simulink model "step1_TrajectoryPlanningModel"  (Simulink 10.2)
settings: Solver=VariableStepAuto  StartTime=0.0  StopTime=10.0  RelTol=1e-3
values from neighbouring files (symbols this model uses):
  L0 = z(7)    [Forward_kinematics.m]    (also in GeometricCalculation_simulink.m = Geoparams(4); PRBDM_3R_parameters.m = 0.03; PRBDM_3R_parameters.mat = 0.03; TrajectoryPlanning_simulink.m = X(8))
  L1 = z(8)    [Forward_kinematics.m]    (also in GeometricCalculation_simulink.m = Geoparams(5); Jacobi.m = x(4); PRBDM_3R_CTC.m = x(19); PRBDM_3R_Dynamic_Matrices_NewtonEular.m = robot_params(4))
  L2 = z(9)    [Forward_kinematics.m]    (also in GeometricCalculation_simulink.m = Geoparams(6); Jacobi.m = x(5); PRBDM_3R_CTC.m = x(20); PRBDM_3R_Dynamic_Matrices_NewtonEular.m = robot_params(5))
  L3 = z(10)    [Forward_kinematics.m]    (also in GeometricCalculation_simulink.m = Geoparams(7); Jacobi.m = x(6); PRBDM_3R_CTC.m = x(21); PRBDM_3R_Dynamic_Matrices_NewtonEular.m = robot_params(6))
  phi = pi/3    (= 1.0471975512)    [PRBDM_3R_test001.m]
  xd = 0.0536    [PRBDM_3R_test001.m]    (also in PRBDM_CTC_task.m = z(13); RRR_CTC_task.m = z(13))
  yd = 0.0135    [PRBDM_3R_test001.m]    (also in PRBDM_CTC_task.m = z(14); RRR_CTC_task.m = z(14))
settings Model: Creator=Master  LastModifiedBy=Master
settings DataIOCC: SaveFormat=Dataset  SignalLoggingSaveFormat=Dataset  ReturnWorkspaceOutputs=on
settings OptimizationCC: LifeSpan=auto
settings DebuggingCC: UnderspecifiedInitializationDetection=Simplified  MergeDetectMultiDrivingBlocksExec=error  FcnCallInpInsideContextMsg=error  SFUnexpectedBacktrackingDiag=error  SFNoUnconditionalDefaultTransitionDiag=error  SFExecutionAtInitializationDiag=warning  UnderSpecifiedDimensionMsg=error  ArithmeticOperatorsInVariantConditions=error
settings HardwareCC: ProdBitPerPointer=64  ProdBitPerSizeT=64  ProdBitPerPtrDiffT=64  ProdLargestAtomicFloat=Float  ProdIntDivRoundTo=Zero  ProdEndianess=LittleEndian  ProdWordSize=64  ProdHWDeviceType=Intel->x86-64 (Windows64)
settings ModelReferenceCC: PropagateSignalLabelsOutOfModel=on
settings SFSimCC: SimUseLocalCustomCode=on  CustomCodeUndefinedFunction=FilterOut
settings RTWCC: RTWUseLocalCustomCode=on
settings CodeAppCC: StateflowObjectComments=off
settings GRTTargetCC: TargetLangStandard=C99 (ISO)  CombineOutputUpdateFcns=on  GRTInterface=off
settings ConfigComp: CovMetricSettings=dwe  CovSaveCumulativeToWorkspaceVar=off  CovSaveSingleToWorkspaceVar=off  CovExternalEMLEnable=on

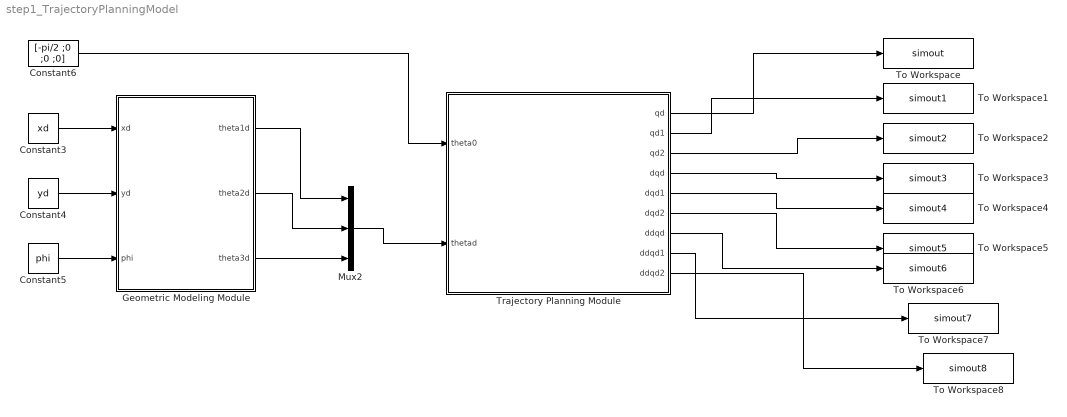
== system step1_TrajectoryPlanningModel ==
  Constant3 : Constant  Value=xd
  Constant4 : Constant  Value=yd
  Constant5 : Constant  Value=phi
  Constant6 : Constant  Value=[-pi/2 ;0 ;0 ;0]
  Geometric Modeling Module : Subsystem
  Mux2 : Mux  Inputs=3
  To Workspace : ToWorkspace  VariableName=simout  SaveFormat=Timeseries  SampleTime=-1
  To Workspace1 : ToWorkspace  VariableName=simout1  SaveFormat=Timeseries  SampleTime=-1
  To Workspace2 : ToWorkspace  VariableName=simout2  SaveFormat=Timeseries  SampleTime=-1
  To Workspace3 : ToWorkspace  VariableName=simout3  SaveFormat=Timeseries  SampleTime=-1
  To Workspace4 : ToWorkspace  VariableName=simout4  SaveFormat=Timeseries  SampleTime=-1
  To Workspace5 : ToWorkspace  VariableName=simout5  SaveFormat=Timeseries  SampleTime=-1
  To Workspace6 : ToWorkspace  VariableName=simout6  SaveFormat=Timeseries  SampleTime=-1
  To Workspace7 : ToWorkspace  VariableName=simout7  SaveFormat=Timeseries  SampleTime=-1
  To Workspace8 : ToWorkspace  VariableName=simout8  SaveFormat=Timeseries  SampleTime=-1
  Trajectory Planning Module : Subsystem
  wires:
  Constant4/1 -> Geometric Modeling Module/2(yd)
  Constant5/1 -> Geometric Modeling Module/3(phi)
  Constant3/1 -> Geometric Modeling Module/1(xd)
  Geometric Modeling Module/1(theta1d) -> Mux2/1
  Geometric Modeling Module/2(theta2d) -> Mux2/2
  Geometric Modeling Module/3(theta3d) -> Mux2/3
  Mux2/1 -> Trajectory Planning Module/2(thetad)
  Constant6/1 -> Trajectory Planning Module/1(theta0)
  Trajectory Planning Module/7(ddqd) -> To Workspace6/1
  Trajectory Planning Module/4(dqd) -> To Workspace3/1
  Trajectory Planning Module/3(qd2) -> To Workspace2/1
  Trajectory Planning Module/5(dqd1) -> To Workspace4/1
  Trajectory Planning Module/2(qd1) -> To Workspace1/1
  Trajectory Planning Module/6(dqd2) -> To Workspace5/1
  Trajectory Planning Module/8(ddqd1) -> To Workspace7/1
  Trajectory Planning Module/9(ddqd2) -> To Workspace8/1
  Trajectory Planning Module/1(qd) -> To Workspace/1

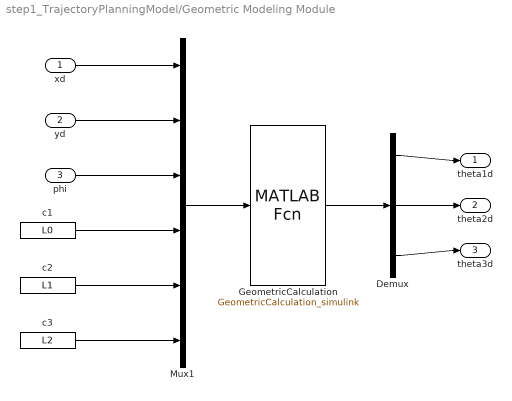
== system step1_TrajectoryPlanningModel/Geometric Modeling Module ==
  xd : Inport
  yd : Inport  Port=2
  phi : Inport  Port=3
  Demux : Demux  Outputs=3
  GeometricCalculation : MATLABFcn  MATLABFcn=GeometricCalculation_simulink
  Mux1 : Mux  Inputs=6
  c1 : Constant  Value=L0
  c2 : Constant  Value=L1
  c3 : Constant  Value=L2
  theta1d : Outport
  theta2d : Outport  Port=2
  theta3d : Outport  Port=3
  wires:
  Mux1/1 -> GeometricCalculation/1
  yd/1 -> Mux1/2
  xd/1 -> Mux1/1
  phi/1 -> Mux1/3
  c1/1 -> Mux1/4
  c3/1 -> Mux1/6
  c2/1 -> Mux1/5
  GeometricCalculation/1 -> Demux/1
  Demux/2 -> theta2d/1
  Demux/1 -> theta1d/1
  Demux/3 -> theta3d/1

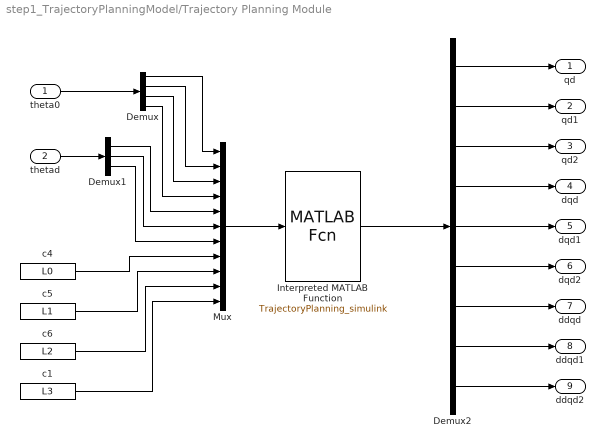
== system step1_TrajectoryPlanningModel/Trajectory Planning Module ==
  theta0 : Inport
  thetad : Inport  Port=2
  Demux : Demux
  Demux1 : Demux  Outputs=3
  Demux2 : Demux  Outputs=9
  Interpreted MATLAB Function : MATLABFcn  MATLABFcn=TrajectoryPlanning_simulink  OutputDimensions=9
  Mux : Mux  Inputs=11
  c1 : Constant  Value=L3
  c4 : Constant  Value=L0
  c5 : Constant  Value=L1
  c6 : Constant  Value=L2
  qd : Outport
  qd1 : Outport  Port=2
  qd2 : Outport  Port=3
  dqd : Outport  Port=4
  dqd1 : Outport  Port=5
  dqd2 : Outport  Port=6
  ddqd : Outport  Port=7
  ddqd1 : Outport  Port=8
  ddqd2 : Outport  Port=9
  wires:
  c4/1 -> Mux/8
  c6/1 -> Mux/10
  c5/1 -> Mux/9
  c1/1 -> Mux/11
  Mux/1 -> Interpreted MATLAB Function/1
  theta0/1 -> Demux/1
  thetad/1 -> Demux1/1
  Demux1/3 -> Mux/7
  Demux1/2 -> Mux/6
  Demux1/1 -> Mux/5
  Demux/4 -> Mux/4
  Demux/3 -> Mux/3
  Demux/2 -> Mux/2
  Demux/1 -> Mux/1
  Interpreted MATLAB Function/1 -> Demux2/1
  Demux2/2 -> qd1/1
  Demux2/9 -> ddqd2/1
  Demux2/1 -> qd/1
  Demux2/3 -> qd2/1
  Demux2/6 -> dqd2/1
  Demux2/5 -> dqd1/1
  Demux2/8 -> ddqd1/1
  Demux2/7 -> ddqd/1
  Demux2/4 -> dqd/1
